simulink model "CP_DTSFC_Lin_a_MainFile_n9945008"  (R2018b)
settings: Solver=VariableStepAuto  StartTime=0.0  StopTime=10.0  RelTol=1e-3
values from neighbouring files (symbols this model uses):
  K_da = place(sysdzoh.A ,sysdzoh.B ,dLambda)    [CP_DTSFC_Lin_a_MainFile_n9945008.m]
  sysdzoh = c2d(sysc,T_s,'zoh')    [CP_DTSFC_Lin_a_MainFile_n9945008.m]    (also in CP_DTSFC_Lin_b_MainFile_n9945008.m)
  T_s = 0.03    [CP_DTSFC_Lin_a_MainFile_n9945008.m]    (also in CP_DTSFC_Lin_b_MainFile_n9945008.m)
  x0 = [0.2 20*pi/180 0 0]'    [CP_DTSFC_Lin_a_MainFile_n9945008.m]    (also in CP_DTSFC_Lin_b_MainFile_n9945008.m)
settings Model: Creator=csmithcripps  LastModifiedBy=csmithcripps

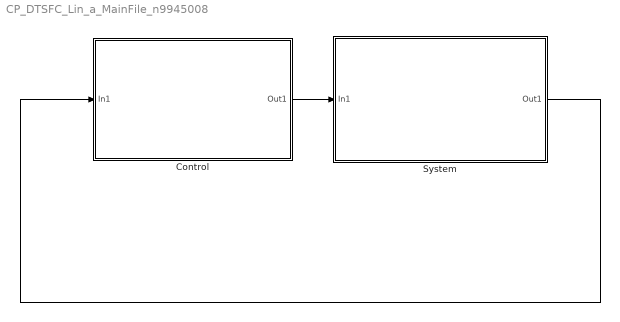
== system CP_DTSFC_Lin_a_MainFile_n9945008 ==
  Control : Subsystem
  "System " : Subsystem
  wires:
  Control/1(Out1) -> "System "/1(In1)
  "System "/1(Out1) -> Control/1(In1)

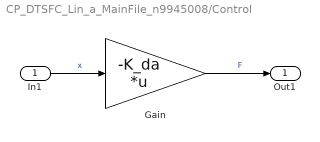
== system CP_DTSFC_Lin_a_MainFile_n9945008/Control ==
  In1 : Inport
  Gain : Gain  Gain=-K_da  Multiplication=Matrix(K*u)
  Out1 : Outport
  wires:
  Gain/1 -> Out1/1  "F"
  In1/1 -> Gain/1  "x"

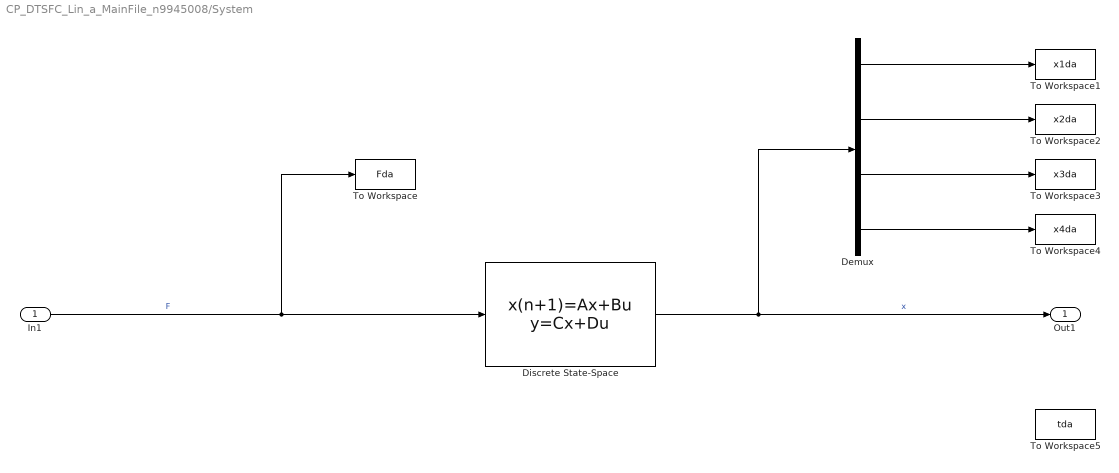
== system CP_DTSFC_Lin_a_MainFile_n9945008/System  ==
  In1 : Inport
  Demux : Demux
  Discrete State-Space : DiscreteStateSpace  A=sysdzoh.A  B=sysdzoh.B  C=sysdzoh.C  D=sysdzoh.D  InitialCondition=x0  SampleTime=T_s
  To Workspace : ToWorkspace  VariableName=Fda  SaveFormat=Timeseries  SampleTime=-1
  To Workspace1 : ToWorkspace  VariableName=x1da  SaveFormat=Timeseries  SampleTime=-1
  To Workspace2 : ToWorkspace  VariableName=x2da  SaveFormat=Timeseries  SampleTime=-1
  To Workspace3 : ToWorkspace  VariableName=x3da  SaveFormat=Timeseries  SampleTime=-1
  To Workspace4 : ToWorkspace  VariableName=x4da  SaveFormat=Timeseries  SampleTime=-1
  To Workspace5 : ToWorkspace  VariableName=tda  SaveFormat=Timeseries  SampleTime=-1
  Out1 : Outport
  wires:
  In1/1 -> To Workspace/1, Discrete State-Space/1  "F"
  Discrete State-Space/1 -> Demux/1, Out1/1  "x"
  Demux/4 -> To Workspace4/1
  Demux/2 -> To Workspace2/1
  Demux/1 -> To Workspace1/1
  Demux/3 -> To Workspace3/1
